simulink library "apm"  (R2021b)
settings: Solver=VariableStepAuto  StartTime=0.0  StopTime=10.0  RelTol=1e-3
settings Model: Creator=FVT22115  LastModifiedBy=FVT23010

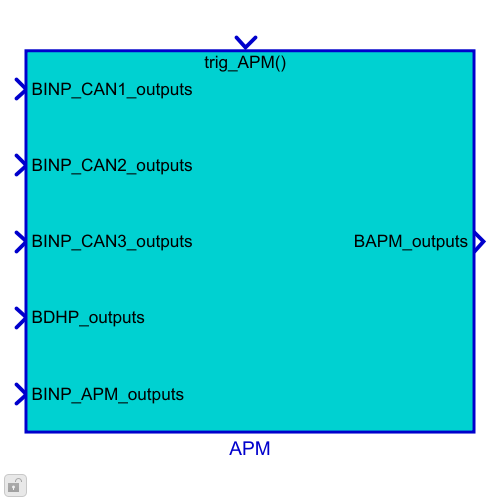
[thumbnail: Simulink's stored preview of the top-level diagram]
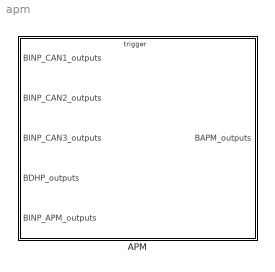
== system apm ==
  APM : Subsystem
      settings: RTWSystemCode=Nonreusable function  RTWFcnNameOpts=Use subsystem name  RTWFileNameOpts=Use subsystem name

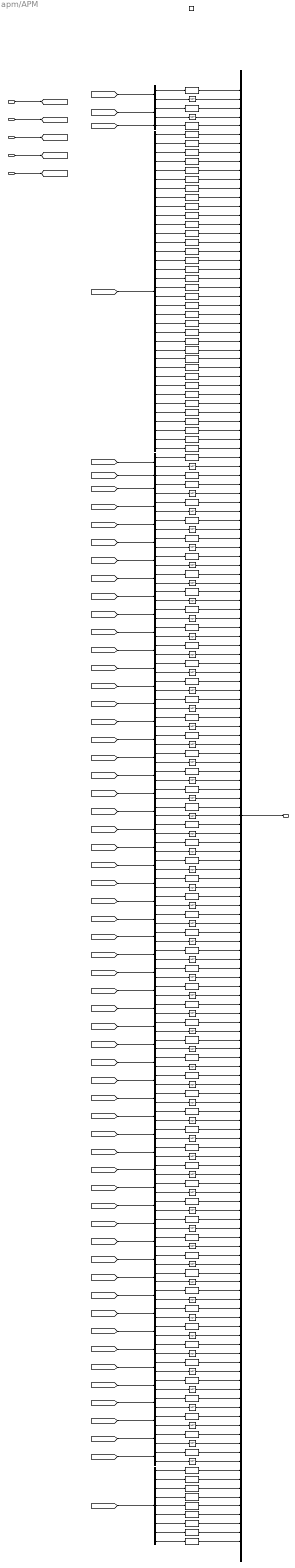
== system apm/APM ==
  BINP_CAN1_outputs : Inport  OutDataTypeStr=Bus: BINP_CAN1_outputs
  BINP_CAN2_outputs : Inport  Port=2  OutDataTypeStr=Bus: BINP_CAN2_outputs
  BINP_CAN3_outputs : Inport  Port=3  OutDataTypeStr=Bus: BINP_CAN3_outputs
  BDHP_outputs : Inport  Port=4  OutDataTypeStr=Bus: BDHP_outputs
  BINP_APM_outputs : Inport  Port=5  OutDataTypeStr=Bus: BINP_APM_outputs
  trig_APM : TriggerPort  TriggerType=function-call  VariantControl=(inherit)
  Bus Creator1 : BusCreator  Inputs=163  OutDataTypeStr=Bus: BAPM_outputs  NonVirtualBus=on
  Bus Selector : BusSelector  OutputSignals=VINP_FSOffSw_enum,VINP_CANMsgValidIVI2_flg
  Bus Selector1 : BusSelector  OutputSignals=VINP_PASDRMR_cm,VINP_PASDRML_cm,VINP_PASDRCR_cm,VINP_PASDRCL_cm,VINP_PASDFMR_cm,VINP_PASDFML_cm,VINP_PASDFCR_cm,VINP_PASDFCL_cm,VINP_APSDRLR_cm,VINP_APSDRLL_cm,VINP_APSDFLR_cm,VINP_APSDFLL_cm,VINP_PASAFCL_enum,VINP_PASARMR_enum,VINP_PASARML_enum,VINP_PASARCR_enum,VINP_PASARCL_enum,VINP_PASAFMR_enum,VINP_PASAFML_enum,VINP_PASAFCR_enum,VINP_USSStaRMR_flg,VINP_USSStaRML_flg,VINP_USSStaRLR_flg,VINP_USSStaRLL_flg,VINP_USSStaRCR_flg,VINP_USSStaRCL_flg,VINP_USSStaFMR_flg,VINP_USSStaFML_flg,VINP_USSStaFLR_flg,VINP_USSStaFLL_flg,VINP_USSStaFCR_flg,VINP_USSStaFCL_flg,VINP_Chime_enum,VINP_SNSRLayout_enum,VINP_StaFSya_flg,VINP_ModOperation_enum
  Bus Selector10 : BusSelector  OutputSignals=VINP_LFRawWhlSpeedV_flg,VINP_CANMsgValidESC1_flg
  Bus Selector11 : BusSelector  OutputSignals=VINP_RFRawWhlSpeedV_flg,VINP_CANMsgValidESC1_flg
  Bus Selector12 : BusSelector  OutputSignals=VINP_LRRawWhlSpeedV_flg,VINP_CANMsgValidESC1_flg
  Bus Selector13 : BusSelector  OutputSignals=VINP_RRRawWhlSpeedV_flg,VINP_CANMsgValidESC1_flg
  Bus Selector14 : BusSelector  OutputSignals=VINP_LFWhlRotDir_enum,VINP_CANMsgValidESC1_flg
  Bus Selector15 : BusSelector  OutputSignals=VINP_RFWhlRotDir_enum,VINP_CANMsgValidESC1_flg
  Bus Selector16 : BusSelector  OutputSignals=VINP_LRWhlRotDir_enum,VINP_CANMsgValidESC1_flg
  Bus Selector17 : BusSelector  OutputSignals=VINP_RRWhlRotDir_enum,VINP_CANMsgValidESC1_flg
  Bus Selector18 : BusSelector  OutputSignals=VINP_LFPulseCountV_flg,VINP_CANMsgValidESC1_flg
  Bus Selector19 : BusSelector  OutputSignals=VINP_RFPulseCountV_flg,VINP_CANMsgValidESC1_flg
  Bus Selector2 : BusSelector  OutputSignals=VINP_VehSpeed_kph,VINP_CANMsgValidESC1_flg
  Bus Selector20 : BusSelector  OutputSignals=VINP_LRPulseCountV_flg,VINP_CANMsgValidESC1_flg
  Bus Selector21 : BusSelector  OutputSignals=VINP_RRPulseCountV_flg,VINP_CANMsgValidESC1_flg
  Bus Selector22 : BusSelector  OutputSignals=VINP_LFPulseCount_enum,VINP_CANMsgValidESC1_flg
  Bus Selector23 : BusSelector  OutputSignals=VINP_RFPulseCount_enum,VINP_CANMsgValidESC1_flg
  Bus Selector24 : BusSelector  OutputSignals=VINP_LRPulseCount_enum,VINP_CANMsgValidESC1_flg
  Bus Selector25 : BusSelector  OutputSignals=VINP_RRPulseCount_enum,VINP_CANMsgValidESC1_flg
  Bus Selector26 : BusSelector  OutputSignals=VINP_ShifterHandleCmd_enum,VINP_CANMsgValidShifter1_flg
  Bus Selector27 : BusSelector  OutputSignals=VINP_DriIntend_enum,VINP_CANMsgValidEPS1_flg
  Bus Selector28 : BusSelector  OutputSignals=VINP_EPSAOIControl_enum,VINP_CANMsgValidEPS1_flg
  Bus Selector29 : BusSelector  OutputSignals=VINP_SASAngle_Deg,VINP_CANMsgValidEPS1_flg
  Bus Selector3 : BusSelector  OutputSignals=VINP_ChrgPlugSta_enum
  Bus Selector30 : BusSelector  OutputSignals=VINP_SASSpeed_degps,VINP_CANMsgValidEPS1_flg
  Bus Selector31 : BusSelector  OutputSignals=VINP_SASSpeedValid_flg,VINP_CANMsgValidEPS1_flg
  Bus Selector32 : BusSelector  OutputSignals=VINP_SASCAL_flg,VINP_CANMsgValidEPS1_flg
  Bus Selector33 : BusSelector  OutputSignals=VINP_SASV_flg,VINP_CANMsgValidEPS1_flg
  Bus Selector34 : BusSelector  OutputSignals=VINP_GRADE_Deg,VINP_CANMsgValidESC1_flg
  Bus Selector35 : BusSelector  OutputSignals=VINP_YawRate_degps,VINP_CANMsgValidESC5_flg
  Bus Selector36 : BusSelector  OutputSignals=VINP_LatAccel_Gps,VINP_CANMsgValidESC5_flg
  Bus Selector37 : BusSelector  OutputSignals=VINP_MCPressure_bar,VINP_CANMsgValidESC5_flg
  Bus Selector38 : BusSelector  OutputSignals=VINP_LongAccel_Gps,VINP_CANMsgValidESC5_flg
  Bus Selector39 : BusSelector  OutputSignals=VINP_YawRateV_flg,VINP_CANMsgValidESC5_flg
  Bus Selector4 : BusSelector  OutputSignals=VINP_BrkPedalPos_pct,VINP_CANMsgValidESC5_flg
  Bus Selector40 : BusSelector  OutputSignals=VINP_LatAccelV_flg,VINP_CANMsgValidESC5_flg
  Bus Selector41 : BusSelector  OutputSignals=VINP_LongAccelV_flg,VINP_CANMsgValidESC5_flg
  Bus Selector42 : BusSelector  OutputSignals=VINP_BrkSwSta_flg,VINP_CANMsgValidESC5_flg
  Bus Selector43 : BusSelector  OutputSignals=VINP_BrkSwV_flg,VINP_CANMsgValidESC5_flg
  Bus Selector44 : BusSelector  OutputSignals=VINP_ESCStandstill_flg,VINP_CANMsgValidESC5_flg
  Bus Selector45 : BusSelector  OutputSignals=VINP_ESCAPSSta_enum,VINP_CANMsgValidESC5_flg
  Bus Selector46 : BusSelector  OutputSignals=VINP_EPBExtReleaseAvail_flg,VINP_CANMsgValidEPB1_flg
  Bus Selector47 : BusSelector  OutputSignals=VINP_EPBExtApplyAvail_flg,VINP_CANMsgValidEPB1_flg
  Bus Selector48 : BusSelector  OutputSignals=VINP_EPBErrSta_enum,VINP_CANMsgValidEPB1_flg
  Bus Selector49 : BusSelector  OutputSignals=VINP_AVMparkingcancel_enum,VINP_CANMsgValidIVI2_flg
  Bus Selector5 : BusSelector  OutputSignals=VDHP_ActAPSPosn_pct
  Bus Selector50 : BusSelector  OutputSignals=VINP_AVMparkingexcute_enum,VINP_CANMsgValidIVI2_flg
  Bus Selector51 : BusSelector  OutputSignals=VINP_AVMParkingmode_enum,VINP_CANMsgValidIVI2_flg
  Bus Selector52 : BusSelector  OutputSignals=VINP_EPBSta_enum,VINP_CANMsgValidEPB1_flg
  Bus Selector53 : BusSelector  OutputSignals=VINP_AVMErrSTA_flg,VINP_CANMsgValidIVI2_flg
  Bus Selector54 : BusSelector  OutputSignals=VINP_IVIStatus_flg,VINP_CANMsgValidIVI2_flg
  Bus Selector55 : BusSelector  OutputSignals=VINP_CAASSw_enum,VINP_CANMsgValidIVI2_flg
  Bus Selector56 : BusSelector  OutputSignals=VINP_IVIScreen_enum,VINP_CANMsgValidIVI2_flg
  Bus Selector57 : BusSelector  OutputSignals=VINP_APSProgressPCT_pct,VINP_APSRQDisplay_enum,VINP_APSSWVer_enum,VINP_APSHWVer_enum,VINP_APSExitCondition_enum,VINP_APSAngleTarget_Deg,VINP_APSVRqEPASCtrl_flg,VINP_APSRqEPASCtrl_flg,VINP_CAASSta_enum
  Bus Selector58 : BusSelector  OutputSignals=VINP_MCPressureV_flg,VINP_CANMsgValidESC5_flg
  Bus Selector59 : BusSelector  OutputSignals=VINP_ABSActive_flg,VINP_CANMsgValidESC1_flg
  Bus Selector6 : BusSelector  OutputSignals=VINP_LFRawWhlSpeed_kph,VINP_CANMsgValidESC1_flg
  Bus Selector61 : BusSelector  OutputSignals=VINP_TCSActive_flg,VINP_CANMsgValidESC1_flg
  Bus Selector62 : BusSelector  OutputSignals=VINP_DriverSeatBeltCmd_flg,VINP_CANMsgValidABM1_flg
  Bus Selector7 : BusSelector  OutputSignals=VINP_RFRawWhlSpeed_kph,VINP_CANMsgValidESC1_flg
  Bus Selector8 : BusSelector  OutputSignals=VINP_LRRawWhlSpeed_kph,VINP_CANMsgValidESC1_flg
  Bus Selector9 : BusSelector  OutputSignals=VINP_RRRawWhlSpeed_kph,VINP_CANMsgValidESC1_flg
  Data Type Conversion{1..104,106} (105 alike) : DataTypeConversion
  Logical Operator{,1..57} (58 alike) : Logic  Operator=NOT  AllPortsSameDT=off  OutDataTypeStr=boolean
  BAPM_outputs : Outport  OutDataTypeStr=Bus: BAPM_outputs
  wires:
  [BINP_CAN2_outputs] -> Bus Selector/1
  [BINP_CAN1_outputs] -> Bus Selector2/1
  Bus Creator1/1 -> BAPM_outputs/1  "BAPM_outputs"
  Bus Selector2/2 -> Logical Operator/1  "<VINP_CANMsgValidESC1_flg>"
  Bus Selector/1 -> Data Type Conversion3/1  "<VINP_FSOffSw_enum>"
  Bus Selector/2 -> Logical Operator1/1  "<VINP_CANMsgValidIVI2_flg>"
  Bus Selector2/1 -> Data Type Conversion1/1  "<VINP_VehSpeed_kph>"
  Bus Selector1/1 -> Data Type Conversion5/1  "<VINP_PASDRMR_cm>"
  Bus Selector1/2 -> Data Type Conversion4/1  "<VINP_PASDRML_cm>"
  Bus Selector1/3 -> Data Type Conversion7/1  "<VINP_PASDRCR_cm>"
  Bus Selector1/4 -> Data Type Conversion6/1  "<VINP_PASDRCL_cm>"
  Bus Selector1/5 -> Data Type Conversion9/1  "<VINP_PASDFMR_cm>"
  Bus Selector1/6 -> Data Type Conversion8/1  "<VINP_PASDFML_cm>"
  Bus Selector1/7 -> Data Type Conversion11/1  "<VINP_PASDFCR_cm>"
  Bus Selector1/8 -> Data Type Conversion10/1  "<VINP_PASDFCL_cm>"
  Bus Selector1/9 -> Data Type Conversion13/1  "<VINP_APSDRLR_cm>"
  Bus Selector1/10 -> Data Type Conversion12/1  "<VINP_APSDRLL_cm>"
  Bus Selector1/11 -> Data Type Conversion15/1  "<VINP_APSDFLR_cm>"
  Bus Selector1/12 -> Data Type Conversion14/1  "<VINP_APSDFLL_cm>"
  Bus Selector1/13 -> Data Type Conversion17/1  "<VINP_PASAFCL_enum>"
  Bus Selector1/14 -> Data Type Conversion16/1  "<VINP_PASARMR_enum>"
  Bus Selector1/15 -> Data Type Conversion25/1  "<VINP_PASARML_enum>"
  Bus Selector1/16 -> Data Type Conversion24/1  "<VINP_PASARCR_enum>"
  Bus Selector1/17 -> Data Type Conversion27/1  "<VINP_PASARCL_enum>"
  Bus Selector1/18 -> Data Type Conversion26/1  "<VINP_PASAFMR_enum>"
  Bus Selector1/19 -> Data Type Conversion29/1  "<VINP_PASAFML_enum>"
  Bus Selector1/20 -> Data Type Conversion28/1  "<VINP_PASAFCR_enum>"
  Bus Selector1/21 -> Data Type Conversion31/1  "<VINP_USSStaRMR_flg>"
  Bus Selector1/22 -> Data Type Conversion30/1  "<VINP_USSStaRML_flg>"
  Bus Selector1/23 -> Data Type Conversion19/1  "<VINP_USSStaRLR_flg>"
  Bus Selector1/24 -> Data Type Conversion18/1  "<VINP_USSStaRLL_flg>"
  Bus Selector1/25 -> Data Type Conversion21/1  "<VINP_USSStaRCR_flg>"
  Bus Selector1/26 -> Data Type Conversion20/1  "<VINP_USSStaRCL_flg>"
  Bus Selector1/27 -> Data Type Conversion23/1  "<VINP_USSStaFMR_flg>"
  Bus Selector1/28 -> Data Type Conversion22/1  "<VINP_USSStaFML_flg>"
  Bus Selector1/29 -> Data Type Conversion39/1  "<VINP_USSStaFLR_flg>"
  Bus Selector1/30 -> Data Type Conversion38/1  "<VINP_USSStaFLL_flg>"
  Bus Selector1/31 -> Data Type Conversion33/1  "<VINP_USSStaFCR_flg>"
  Bus Selector1/32 -> Data Type Conversion32/1  "<VINP_USSStaFCL_flg>"
  Bus Selector1/33 -> Data Type Conversion35/1  "<VINP_Chime_enum>"
  Bus Selector1/34 -> Data Type Conversion34/1  "<VINP_SNSRLayout_enum>"
  Bus Selector1/35 -> Data Type Conversion37/1  "<VINP_StaFSya_flg>"
  Bus Selector1/36 -> Data Type Conversion36/1  "<VINP_ModOperation_enum>"
  Data Type Conversion1/1 -> Bus Creator1/1  "VAPM_VehSpeed_kph"
  Logical Operator/1 -> Bus Creator1/2  "VAPM_VehSpeedTimeOut_flg"
  Data Type Conversion3/1 -> Bus Creator1/3  "VAPM_FSOffSw_enum"
  Logical Operator1/1 -> Bus Creator1/4  "VAPM_FSOffSwTimeOut_flg"
  Bus Selector3/1 -> Data Type Conversion2/1  "<VINP_ChrgPlugSta_enum>"
  Data Type Conversion2/1 -> Bus Creator1/5  "VAPM_ChrgPlugSta_enum"
  BINP_CAN1_outputs/1 -> [BINP_CAN1_outputs]  "BINP_CAN1_outputs"
  BINP_CAN2_outputs/1 -> [BINP_CAN2_outputs]  "BINP_CAN2_outputs"
  BINP_CAN3_outputs/1 -> [BINP_CAN3_outputs]  "BINP_CAN3_outputs"
  [BINP_CAN1_outputs] -> Bus Selector4/1
  Bus Selector4/1 -> Data Type Conversion40/1  "<VINP_BrkPedalPos_pct>"
  Bus Selector4/2 -> Logical Operator2/1  "<VINP_CANMsgValidESC5_flg>"
  [BDHP_outputs] -> Bus Selector5/1
  BDHP_outputs/1 -> [BDHP_outputs]  "BDHP_outputs"
  Bus Selector6/1 -> Data Type Conversion42/1  "<VINP_LFRawWhlSpeed_kph>"
  [BINP_CAN1_outputs] -> Bus Selector6/1
  Bus Selector6/2 -> Logical Operator3/1  "<VINP_CANMsgValidESC1_flg>"
  Bus Selector7/2 -> Logical Operator4/1  "<VINP_CANMsgValidESC1_flg>"
  [BINP_CAN1_outputs] -> Bus Selector7/1
  Bus Selector7/1 -> Data Type Conversion43/1  "<VINP_RFRawWhlSpeed_kph>"
  Bus Selector8/1 -> Data Type Conversion44/1  "<VINP_LRRawWhlSpeed_kph>"
  [BINP_CAN1_outputs] -> Bus Selector8/1
  Bus Selector8/2 -> Logical Operator5/1  "<VINP_CANMsgValidESC1_flg>"
  Bus Selector9/2 -> Logical Operator6/1  "<VINP_CANMsgValidESC1_flg>"
  [BINP_CAN1_outputs] -> Bus Selector9/1
  Bus Selector9/1 -> Data Type Conversion45/1  "<VINP_RRRawWhlSpeed_kph>"
  [BINP_CAN1_outputs] -> Bus Selector13/1
  [BINP_CAN1_outputs] -> Bus Selector12/1
  [BINP_CAN1_outputs] -> Bus Selector11/1
  [BINP_CAN1_outputs] -> Bus Selector10/1
  Bus Selector14/1 -> Data Type Conversion50/1  "<VINP_LFWhlRotDir_enum>"
  [BINP_CAN1_outputs] -> Bus Selector14/1
  Bus Selector14/2 -> Logical Operator12/1  "<VINP_CANMsgValidESC1_flg>"
  Bus Selector15/2 -> Logical Operator13/1  "<VINP_CANMsgValidESC1_flg>"
  [BINP_CAN1_outputs] -> Bus Selector15/1
  Bus Selector15/1 -> Data Type Conversion51/1  "<VINP_RFWhlRotDir_enum>"
  Bus Selector16/1 -> Data Type Conversion52/1  "<VINP_LRWhlRotDir_enum>"
  [BINP_CAN1_outputs] -> Bus Selector16/1
  Bus Selector16/2 -> Logical Operator14/1  "<VINP_CANMsgValidESC1_flg>"
  Bus Selector17/2 -> Logical Operator11/1  "<VINP_CANMsgValidESC1_flg>"
  [BINP_CAN1_outputs] -> Bus Selector17/1
  Bus Selector17/1 -> Data Type Conversion53/1  "<VINP_RRWhlRotDir_enum>"
  Bus Selector21/1 -> Data Type Conversion57/1  "<VINP_RRPulseCountV_flg>"
  [BINP_CAN1_outputs] -> Bus Selector21/1
  Bus Selector21/2 -> Logical Operator15/1  "<VINP_CANMsgValidESC1_flg>"
  Bus Selector20/2 -> Logical Operator18/1  "<VINP_CANMsgValidESC1_flg>"
  [BINP_CAN1_outputs] -> Bus Selector20/1
  Bus Selector20/1 -> Data Type Conversion56/1  "<VINP_LRPulseCountV_flg>"
  Bus Selector19/1 -> Data Type Conversion55/1  "<VINP_RFPulseCountV_flg>"
  [BINP_CAN1_outputs] -> Bus Selector19/1
  Bus Selector19/2 -> Logical Operator17/1  "<VINP_CANMsgValidESC1_flg>"
  Bus Selector18/2 -> Logical Operator16/1  "<VINP_CANMsgValidESC1_flg>"
  [BINP_CAN1_outputs] -> Bus Selector18/1
  Bus Selector18/1 -> Data Type Conversion54/1  "<VINP_LFPulseCountV_flg>"
  Bus Selector5/1 -> Data Type Conversion41/1  "<VDHP_ActAPSPosn_pct>"
  [BINP_CAN3_outputs] -> Bus Selector3/1
  Data Type Conversion5/1 -> Bus Creator1/6  "VAPM_PASDRMR_cm"
  Data Type Conversion4/1 -> Bus Creator1/7  "VAPM_PASDRML_cm"
  Data Type Conversion7/1 -> Bus Creator1/8  "VAPM_PASDRCR_cm"
  Data Type Conversion6/1 -> Bus Creator1/9  "VAPM_PASDRCL_cm"
  Data Type Conversion9/1 -> Bus Creator1/10  "VAPM_PASDFMR_cm"
  Data Type Conversion8/1 -> Bus Creator1/11  "VAPM_PASDFML_cm"
  Data Type Conversion11/1 -> Bus Creator1/12  "VAPM_PASDFCR_cm"
  Data Type Conversion10/1 -> Bus Creator1/13  "VAPM_PASDFCL_cm"
  Data Type Conversion13/1 -> Bus Creator1/14  "VAPM_APSDRLR_cm"
  Data Type Conversion12/1 -> Bus Creator1/15  "VAPM_APSDRLL_cm"
  Data Type Conversion15/1 -> Bus Creator1/16  "VAPM_APSDFLR_cm"
  Data Type Conversion14/1 -> Bus Creator1/17  "VAPM_APSDFLL_cm"
  Data Type Conversion17/1 -> Bus Creator1/18  "VAPM_PASAFCL_enum"
  Data Type Conversion16/1 -> Bus Creator1/19  "VAPM_PASARMR_enum"
  Data Type Conversion25/1 -> Bus Creator1/20  "VAPM_PASARML_enum"
  Data Type Conversion24/1 -> Bus Creator1/21  "VAPM_PASARCR_enum"
  Data Type Conversion27/1 -> Bus Creator1/22  "VAPM_PASARCL_enum"
  Data Type Conversion26/1 -> Bus Creator1/23  "VAPM_PASAFMR_enum"
  Data Type Conversion29/1 -> Bus Creator1/24  "VAPM_PASAFML_enum"
  Data Type Conversion28/1 -> Bus Creator1/25  "VAPM_PASAFCR_enum"
  Data Type Conversion31/1 -> Bus Creator1/26  "VAPM_USSStaRMR_flg"
  Data Type Conversion30/1 -> Bus Creator1/27  "VAPM_USSStaRML_flg"
  Data Type Conversion19/1 -> Bus Creator1/28  "VAPM_USSStaRLR_flg"
  Data Type Conversion18/1 -> Bus Creator1/29  "VAPM_USSStaRLL_flg"
  Data Type Conversion21/1 -> Bus Creator1/30  "VAPM_USSStaRCR_flg"
  Data Type Conversion20/1 -> Bus Creator1/31  "VAPM_USSStaRCL_flg"
  Data Type Conversion23/1 -> Bus Creator1/32  "VAPM_USSStaFMR_flg"
  Data Type Conversion22/1 -> Bus Creator1/33  "VAPM_USSStaFML_flg"
  Data Type Conversion39/1 -> Bus Creator1/34  "VAPM_USSStaFLR_flg"
  Data Type Conversion38/1 -> Bus Creator1/35  "VAPM_USSStaFLL_flg"
  Data Type Conversion33/1 -> Bus Creator1/36  "VAPM_USSStaFCR_flg"
  Data Type Conversion32/1 -> Bus Creator1/37  "VAPM_USSStaFCL_flg"
  Data Type Conversion35/1 -> Bus Creator1/38  "VAPM_Chime_enum"
  Data Type Conversion34/1 -> Bus Creator1/39  "VAPM_SNSRLayout_enum"
  Data Type Conversion37/1 -> Bus Creator1/40  "VAPM_StaFSya_flg"
  Data Type Conversion36/1 -> Bus Creator1/41  "VAPM_ModOperation_enum"
  Data Type Conversion40/1 -> Bus Creator1/42  "VAPM_BrkPedalPos_pct"
  Data Type Conversion41/1 -> Bus Creator1/44  "VAPM_ActAPSPosn_pct"
  Data Type Conversion42/1 -> Bus Creator1/45  "VAPM_LFRawWhlSpeed_kph"
  Data Type Conversion43/1 -> Bus Creator1/47  "VAPM_RFRawWhlSpeed_kph"
  Data Type Conversion44/1 -> Bus Creator1/49  "VAPM_LRRawWhlSpeed_kph"
  Data Type Conversion45/1 -> Bus Creator1/51  "VAPM_RRRawWhlSpeed_kph"
  Data Type Conversion46/1 -> Bus Creator1/53  "VAPM_LFRawWhlSpeedV_flg"
  Data Type Conversion47/1 -> Bus Creator1/55  "VAPM_RFRawWhlSpeedV_flg"
  Data Type Conversion48/1 -> Bus Creator1/57  "VAPM_LRRawWhlSpeedV_flg"
  Data Type Conversion49/1 -> Bus Creator1/59  "VAPM_RRRawWhlSpeedV_flg"
  Data Type Conversion50/1 -> Bus Creator1/61  "VAPM_LFWhlRotDir_enum"
  Data Type Conversion51/1 -> Bus Creator1/63  "VAPM_RFWhlRotDir_enum"
  Data Type Conversion52/1 -> Bus Creator1/65  "VAPM_LRWhlRotDir_enum"
  Data Type Conversion53/1 -> Bus Creator1/67  "VAPM_RRWhlRotDir_enum"
  Data Type Conversion54/1 -> Bus Creator1/69  "VAPM_LFPulseCountV_flg"
  Data Type Conversion55/1 -> Bus Creator1/71  "VAPM_RFPulseCountV_flg"
  Data Type Conversion56/1 -> Bus Creator1/73  "VAPM_LRPulseCountV_flg"
  Data Type Conversion57/1 -> Bus Creator1/75  "VAPM_RRPulseCountV_flg"
  Logical Operator2/1 -> Bus Creator1/43  "VAPM_BrkPedalPosTimeOut_flg"
  Logical Operator3/1 -> Bus Creator1/46  "VAPM_LFRawWhlSpeedTimeOut_flg"
  Logical Operator4/1 -> Bus Creator1/48  "VAPM_RFRawWhlSpeedTimeOut_flg"
  Logical Operator5/1 -> Bus Creator1/50  "VAPM_LRRawWhlSpeedTimeOut_flg"
  Logical Operator6/1 -> Bus Creator1/52  "VAPM_RRRawWhlSpeedTimeOut_flg"
  Logical Operator7/1 -> Bus Creator1/54  "VAPM_LFRawWhlSpeedVTimeOut_flg"
  Logical Operator8/1 -> Bus Creator1/56  "VAPM_RFRawWhlSpeedVTimeOut_flg"
  Logical Operator9/1 -> Bus Creator1/58  "VAPM_LRRawWhlSpeedVTimeOut_flg"
  Logical Operator10/1 -> Bus Creator1/60  "VAPM_RRRawWhlSpeedVTimeOut_flg"
  Logical Operator12/1 -> Bus Creator1/62  "VAPM_LFWhlRotDirTimeOut_flg"
  Logical Operator13/1 -> Bus Creator1/64  "VAPM_RFWhlRotDirTimeOut_flg"
  Logical Operator14/1 -> Bus Creator1/66  "VAPM_LRWhlRotDirTimeOut_flg"
  Logical Operator11/1 -> Bus Creator1/68  "VAPM_RRWhlRotDirTimeOut_flg"
  Logical Operator16/1 -> Bus Creator1/70  "VAPM_LFPulseCountVTimeOut_flg"
  Logical Operator17/1 -> Bus Creator1/72  "VAPM_RFPulseCountVTimeOut_flg"
  Logical Operator18/1 -> Bus Creator1/74  "VAPM_LRPulseCountVTimeOut_flg"
  Logical Operator15/1 -> Bus Creator1/76  "VAPM_RRPulseCountVTimeOut_flg"
  Logical Operator19/1 -> Bus Creator1/84  "VAPM_RRPulseCountTimeOut_flg"
  Logical Operator22/1 -> Bus Creator1/82  "VAPM_LRPulseCountTimeOut_flg"
  Logical Operator21/1 -> Bus Creator1/80  "VAPM_RFPulseCountTimeOut_flg"
  Logical Operator20/1 -> Bus Creator1/78  "VAPM_LFPulseCountTimeOut_flg"
  Data Type Conversion61/1 -> Bus Creator1/83  "VAPM_RRPulseCount_enum"
  Data Type Conversion60/1 -> Bus Creator1/81  "VAPM_LRPulseCount_enum"
  Data Type Conversion59/1 -> Bus Creator1/79  "VAPM_RFPulseCount_enum"
  Data Type Conversion58/1 -> Bus Creator1/77  "VAPM_LFPulseCount_enum"
  Bus Selector22/1 -> Data Type Conversion58/1  "<VINP_LFPulseCount_enum>"
  [BINP_CAN1_outputs] -> Bus Selector22/1
  Bus Selector22/2 -> Logical Operator20/1  "<VINP_CANMsgValidESC1_flg>"
  Bus Selector23/2 -> Logical Operator21/1  "<VINP_CANMsgValidESC1_flg>"
  [BINP_CAN1_outputs] -> Bus Selector23/1
  Bus Selector23/1 -> Data Type Conversion59/1  "<VINP_RFPulseCount_enum>"
  Bus Selector24/1 -> Data Type Conversion60/1  "<VINP_LRPulseCount_enum>"
  [BINP_CAN1_outputs] -> Bus Selector24/1
  Bus Selector24/2 -> Logical Operator22/1  "<VINP_CANMsgValidESC1_flg>"
  Bus Selector25/2 -> Logical Operator19/1  "<VINP_CANMsgValidESC1_flg>"
  [BINP_CAN1_outputs] -> Bus Selector25/1
  Bus Selector25/1 -> Data Type Conversion61/1  "<VINP_RRPulseCount_enum>"
  [BINP_CAN3_outputs] -> Bus Selector26/1
  Bus Selector26/1 -> Data Type Conversion62/1  "<VINP_ShifterHandleCmd_enum>"
  Bus Selector26/2 -> Logical Operator23/1  "<VINP_CANMsgValidShifter1_flg>"
  Data Type Conversion62/1 -> Bus Creator1/85  "VAPM_ShifterHandleCmd_enum"
  Logical Operator23/1 -> Bus Creator1/86  "VAPM_ShifterHandleCmdTimeOut_flg"
  [BINP_CAN1_outputs] -> Bus Selector27/1
  [BINP_CAN1_outputs] -> Bus Selector28/1
  [BINP_CAN1_outputs] -> Bus Selector29/1
  Bus Selector29/1 -> Data Type Conversion65/1  "<VINP_SASAngle_Deg>"
  Bus Selector29/2 -> Logical Operator26/1  "<VINP_CANMsgValidEPS1_flg>"
  Bus Selector30/2 -> Logical Operator27/1  "<VINP_CANMsgValidEPS1_flg>"
  [BINP_CAN1_outputs] -> Bus Selector30/1
  [BINP_CAN1_outputs] -> Bus Selector31/1
  Bus Selector31/2 -> Logical Operator28/1  "<VINP_CANMsgValidEPS1_flg>"
  Data Type Conversion65/1 -> Bus Creator1/91  "VAPM_SASAngle_Deg"
  Logical Operator26/1 -> Bus Creator1/92  "VAPM_SASAngleTimeOut_flg"
  Bus Selector32/2 -> Logical Operator29/1  "<VINP_CANMsgValidEPS1_flg>"
  [BINP_CAN1_outputs] -> Bus Selector32/1
  [BINP_CAN1_outputs] -> Bus Selector33/1
  Bus Selector33/2 -> Logical Operator30/1  "<VINP_CANMsgValidEPS1_flg>"
  Logical Operator31/1 -> Bus Creator1/102  "VAPM_GRADETimeOut_flg"
  Data Type Conversion70/1 -> Bus Creator1/101  "VAPM_GRADE_Deg"
  Bus Selector34/2 -> Logical Operator31/1  "<VINP_CANMsgValidESC1_flg>"
  Bus Selector34/1 -> Data Type Conversion70/1  "<VINP_GRADE_Deg>"
  [BINP_CAN1_outputs] -> Bus Selector34/1
  [BINP_CAN1_outputs] -> Bus Selector35/1
  Bus Selector35/1 -> Data Type Conversion71/1  "<VINP_YawRate_degps>"
  Bus Selector35/2 -> Logical Operator32/1  "<VINP_CANMsgValidESC5_flg>"
  Data Type Conversion71/1 -> Bus Creator1/103  "VAPM_YawRate_degps"
  Logical Operator32/1 -> Bus Creator1/104  "VAPM_YawRateTimeOut_flg"
  Logical Operator33/1 -> Bus Creator1/106  "VAPM_LatAccelTimeOut_flg"
  Data Type Conversion72/1 -> Bus Creator1/105  "VAPM_LatAccel_Gps"
  Bus Selector36/2 -> Logical Operator33/1  "<VINP_CANMsgValidESC5_flg>"
  Bus Selector36/1 -> Data Type Conversion72/1  "<VINP_LatAccel_Gps>"
  [BINP_CAN1_outputs] -> Bus Selector36/1
  [BINP_CAN1_outputs] -> Bus Selector37/1
  Bus Selector37/1 -> Data Type Conversion73/1  "<VINP_MCPressure_bar>"
  Bus Selector37/2 -> Logical Operator34/1  "<VINP_CANMsgValidESC5_flg>"
  Bus Selector38/2 -> Logical Operator35/1  "<VINP_CANMsgValidESC5_flg>"
  Bus Selector38/1 -> Data Type Conversion74/1  "<VINP_LongAccel_Gps>"
  [BINP_CAN1_outputs] -> Bus Selector38/1
  Data Type Conversion74/1 -> Bus Creator1/107  "VAPM_LongAccel_Gps"
  Logical Operator35/1 -> Bus Creator1/108  "VAPM_LongAccelTimeOut_flg"
  Data Type Conversion73/1 -> Bus Creator1/109  "VAPM_MCPressure_bar"
  Logical Operator34/1 -> Bus Creator1/110  "VAPM_MCPressureTimeOut_flg"
  [BINP_CAN1_outputs] -> Bus Selector41/1
  Bus Selector41/2 -> Logical Operator38/1  "<VINP_CANMsgValidESC5_flg>"
  [BINP_CAN1_outputs] -> Bus Selector40/1
  Bus Selector40/2 -> Logical Operator37/1  "<VINP_CANMsgValidESC5_flg>"
  Bus Selector39/2 -> Logical Operator36/1  "<VINP_CANMsgValidESC5_flg>"
  [BINP_CAN1_outputs] -> Bus Selector39/1
  Bus Selector42/2 -> Logical Operator39/1  "<VINP_CANMsgValidESC5_flg>"
  [BINP_CAN1_outputs] -> Bus Selector42/1
  Bus Selector42/1 -> Data Type Conversion78/1  "<VINP_BrkSwSta_flg>"
  Data Type Conversion78/1 -> Bus Creator1/119  "VAPM_BrkSwSta_flg"
  Logical Operator39/1 -> Bus Creator1/120  "VAPM_BrkSwStaTimeOut_flg"
  Logical Operator40/1 -> Bus Creator1/122  "VAPM_BrkSwVTimeOut_flg"
  Data Type Conversion79/1 -> Bus Creator1/121  "VAPM_BrkSwV_flg"
  Bus Selector43/1 -> Data Type Conversion79/1  "<VINP_BrkSwV_flg>"
  [BINP_CAN1_outputs] -> Bus Selector43/1
  Bus Selector43/2 -> Logical Operator40/1  "<VINP_CANMsgValidESC5_flg>"
  [BINP_CAN1_outputs] -> Bus Selector44/1
  Bus Selector44/2 -> Logical Operator41/1  "<VINP_CANMsgValidESC5_flg>"
  Bus Selector45/2 -> Logical Operator42/1  "<VINP_CANMsgValidESC5_flg>"
  [BINP_CAN1_outputs] -> Bus Selector45/1
  [BINP_CAN1_outputs] -> Bus Selector47/1
  Bus Selector47/2 -> Logical Operator44/1  "<VINP_CANMsgValidEPB1_flg>"
  Bus Selector46/2 -> Logical Operator43/1  "<VINP_CANMsgValidEPB1_flg>"
  [BINP_CAN1_outputs] -> Bus Selector46/1
  Bus Selector48/2 -> Logical Operator45/1  "<VINP_CANMsgValidEPB1_flg>"
  [BINP_CAN1_outputs] -> Bus Selector48/1
  Bus Selector48/1 -> Data Type Conversion84/1  "<VINP_EPBErrSta_enum>"
  Data Type Conversion84/1 -> Bus Creator1/131  "VAPM_EPBErrSta_enum"
  Logical Operator45/1 -> Bus Creator1/132  "VAPM_EPBErrStaTimeOut_flg"
  Bus Selector49/2 -> Logical Operator46/1  "<VINP_CANMsgValidIVI2_flg>"
  [BINP_CAN2_outputs] -> Bus Selector49/1
  [BINP_CAN2_outputs] -> Bus Selector50/1
  Bus Selector50/2 -> Logical Operator47/1  "<VINP_CANMsgValidIVI2_flg>"
  Bus Selector51/2 -> Logical Operator48/1  "<VINP_CANMsgValidIVI2_flg>"
  [BINP_CAN2_outputs] -> Bus Selector51/1
  Logical Operator49/1 -> Bus Creator1/134  "VAPM_EPBStaTimeOut_flg"
  Data Type Conversion88/1 -> Bus Creator1/133  "VAPM_EPBSta_enum"
  Bus Selector52/1 -> Data Type Conversion88/1  "<VINP_EPBSta_enum>"
  [BINP_CAN1_outputs] -> Bus Selector52/1
  Bus Selector52/2 -> Logical Operator49/1  "<VINP_CANMsgValidEPB1_flg>"
  [BINP_CAN2_outputs] -> Bus Selector53/1
  Bus Selector53/2 -> Logical Operator50/1  "<VINP_CANMsgValidIVI2_flg>"
  Bus Selector54/2 -> Logical Operator51/1  "<VINP_CANMsgValidIVI2_flg>"
  [BINP_CAN2_outputs] -> Bus Selector54/1
  Bus Selector54/1 -> Data Type Conversion90/1  "<VINP_IVIStatus_flg>"
  Data Type Conversion90/1 -> Bus Creator1/143  "VAPM_IVIStatus_flg"
  Logical Operator51/1 -> Bus Creator1/144  "VAPM_IVIStatusTimeOut_flg"
  [BINP_CAN2_outputs] -> Bus Selector55/1
  Bus Selector55/2 -> Logical Operator52/1  "<VINP_CANMsgValidIVI2_flg>"
  Bus Selector56/2 -> Logical Operator53/1  "<VINP_CANMsgValidIVI2_flg>"
  [BINP_CAN2_outputs] -> Bus Selector56/1
  Logical Operator27/1 -> Bus Creator1/94  "VAPM_SASSpeedTimeOut_flg"
  Logical Operator24/1 -> Bus Creator1/88  "VAPM_DriIntendTimeOut_flg"
  Logical Operator25/1 -> Bus Creator1/90  "VAPM_EPSAOIControlTimeOut_flg"
  Logical Operator28/1 -> Bus Creator1/96  "VAPM_SASSpeedValidTimeOut_flg"
  Logical Operator29/1 -> Bus Creator1/98  "VAPM_SASCALTimeOut_flg"
  Logical Operator30/1 -> Bus Creator1/100  "VAPM_SASVTimeOut_flg"
  Logical Operator36/1 -> Bus Creator1/112  "VAPM_YawRateVTimeOut_flg"
  Logical Operator37/1 -> Bus Creator1/114  "VAPM_LatAccelVTimeOut_flg"
  Logical Operator38/1 -> Bus Creator1/116  "VAPM_LongAccelVTimeOut_flg"
  Logical Operator41/1 -> Bus Creator1/124  "VAPM_ESCStandstillTimeOut_flg"
  Logical Operator42/1 -> Bus Creator1/126  "VAPM_ESCAPSStaTimeOut_flg"
  Logical Operator43/1 -> Bus Creator1/128  "VAPM_EPBExtReleaseAvailTimeOut_flg"
  Logical Operator44/1 -> Bus Creator1/130  "VAPM_EPBExtApplyAvailTimeOut_flg"
  Logical Operator46/1 -> Bus Creator1/136  "VAPM_AVMparkingcancelTimeOut_flg"
  Logical Operator47/1 -> Bus Creator1/138  "VAPM_AVMparkingexcuteTimeOut_flg"
  Logical Operator48/1 -> Bus Creator1/140  "VAPM_AVMParkingmodeTimeOut_flg"
  Logical Operator50/1 -> Bus Creator1/142  "VAPM_AVMErrSTATimeOut_flg"
  Logical Operator52/1 -> Bus Creator1/146  "VAPM_CAASSwTimeOut_flg"
  Logical Operator53/1 -> Bus Creator1/148  "VAPM_IVIScreenTimeOut_flg"
  BINP_APM_outputs/1 -> [BINP_APM_outputs]  "BINP_APM_outputs"
  [BINP_APM_outputs] -> Bus Selector1/1
  [BINP_APM_outputs] -> Bus Selector57/1
  Bus Selector57/9 -> Data Type Conversion101/1  "<VINP_CAASSta_enum>"
  Bus Selector57/8 -> Data Type Conversion102/1  "<VINP_APSRqEPASCtrl_flg>"
  Bus Selector57/7 -> Data Type Conversion100/1  "<VINP_APSVRqEPASCtrl_flg>"
  Bus Selector57/6 -> Data Type Conversion98/1  "<VINP_APSAngleTarget_Deg>"
  Bus Selector57/5 -> Data Type Conversion97/1  "<VINP_APSExitCondition_enum>"
  Bus Selector57/4 -> Data Type Conversion96/1  "<VINP_APSHWVer_enum>"
  Bus Selector57/3 -> Data Type Conversion95/1  "<VINP_APSSWVer_enum>"
  Bus Selector57/2 -> Data Type Conversion94/1  "<VINP_APSRQDisplay_enum>"
  Bus Selector57/1 -> Data Type Conversion93/1  "<VINP_APSProgressPCT_pct>"
  Bus Selector27/1 -> Data Type Conversion63/1  "<VINP_DriIntend_enum>"
  Data Type Conversion63/1 -> Bus Creator1/87  "VAPM_DriIntend_enum"
  Bus Selector27/2 -> Logical Operator24/1  "<VINP_CANMsgValidEPS1_flg>"
  Bus Selector28/1 -> Data Type Conversion64/1  "<VINP_EPSAOIControl_enum>"
  Data Type Conversion64/1 -> Bus Creator1/89  "VAPM_EPSAOIControl_enum"
  Bus Selector30/1 -> Data Type Conversion66/1  "<VINP_SASSpeed_degps>"
  Data Type Conversion66/1 -> Bus Creator1/93  "VAPM_SASSpeed_degps"
  Bus Selector31/1 -> Data Type Conversion67/1  "<VINP_SASSpeedValid_flg>"
  Data Type Conversion67/1 -> Bus Creator1/95  "VAPM_SASSpeedValid_flg"
  Bus Selector32/1 -> Data Type Conversion68/1  "<VINP_SASCAL_flg>"
  Data Type Conversion68/1 -> Bus Creator1/97  "VAPM_SASCAL_flg"
  Bus Selector33/1 -> Data Type Conversion69/1  "<VINP_SASV_flg>"
  Data Type Conversion69/1 -> Bus Creator1/99  "VAPM_SASV_flg"
  Bus Selector39/1 -> Data Type Conversion75/1  "<VINP_YawRateV_flg>"
  Data Type Conversion75/1 -> Bus Creator1/111  "VAPM_YawRateV_flg"
  Bus Selector40/1 -> Data Type Conversion76/1  "<VINP_LatAccelV_flg>"
  Data Type Conversion76/1 -> Bus Creator1/113  "VAPM_LatAccelV_flg"
  Bus Selector41/1 -> Data Type Conversion77/1  "<VINP_LongAccelV_flg>"
  Data Type Conversion77/1 -> Bus Creator1/115  "VAPM_LongAccelV_flg"
  Bus Selector44/1 -> Data Type Conversion80/1  "<VINP_ESCStandstill_flg>"
  Data Type Conversion80/1 -> Bus Creator1/123  "VAPM_ESCStandstill_flg"
  Bus Selector45/1 -> Data Type Conversion81/1  "<VINP_ESCAPSSta_enum>"
  Data Type Conversion81/1 -> Bus Creator1/125  "VAPM_ESCAPSSta_enum"
  Bus Selector46/1 -> Data Type Conversion82/1  "<VINP_EPBExtReleaseAvail_flg>"
  Data Type Conversion82/1 -> Bus Creator1/127  "VAPM_EPBExtReleaseAvail_flg"
  Bus Selector47/1 -> Data Type Conversion83/1  "<VINP_EPBExtApplyAvail_flg>"
  Data Type Conversion83/1 -> Bus Creator1/129  "VAPM_EPBExtApplyAvail_flg"
  Bus Selector49/1 -> Data Type Conversion85/1  "<VINP_AVMparkingcancel_enum>"
  Data Type Conversion85/1 -> Bus Creator1/135  "VAPM_AVMparkingcancel_enum"
  Bus Selector50/1 -> Data Type Conversion86/1  "<VINP_AVMparkingexcute_enum>"
  Data Type Conversion86/1 -> Bus Creator1/137  "VAPM_AVMparkingexcute_enum"
  Bus Selector51/1 -> Data Type Conversion87/1  "<VINP_AVMParkingmode_enum>"
  Data Type Conversion87/1 -> Bus Creator1/139  "VAPM_AVMParkingmode_enum"
  Bus Selector53/1 -> Data Type Conversion89/1  "<VINP_AVMErrSTA_flg>"
  Data Type Conversion89/1 -> Bus Creator1/141  "VAPM_AVMErrSTA_flg"
  Bus Selector55/1 -> Data Type Conversion91/1  "<VINP_CAASSw_enum>"
  Data Type Conversion91/1 -> Bus Creator1/145  "VAPM_CAASSw_enum"
  Bus Selector56/1 -> Data Type Conversion92/1  "<VINP_IVIScreen_enum>"
  Data Type Conversion92/1 -> Bus Creator1/147  "VAPM_IVIScreen_enum"
  Bus Selector10/1 -> Data Type Conversion46/1  "<VINP_LFRawWhlSpeedV_flg>"
  Bus Selector10/2 -> Logical Operator7/1  "<VINP_CANMsgValidESC1_flg>"
  Bus Selector11/1 -> Data Type Conversion47/1  "<VINP_RFRawWhlSpeedV_flg>"
  Bus Selector11/2 -> Logical Operator8/1  "<VINP_CANMsgValidESC1_flg>"
  Bus Selector12/1 -> Data Type Conversion48/1  "<VINP_LRRawWhlSpeedV_flg>"
  Bus Selector12/2 -> Logical Operator9/1  "<VINP_CANMsgValidESC1_flg>"
  Bus Selector13/1 -> Data Type Conversion49/1  "<VINP_RRRawWhlSpeedV_flg>"
  Bus Selector13/2 -> Logical Operator10/1  "<VINP_CANMsgValidESC1_flg>"
  Bus Selector58/1 -> Data Type Conversion106/1  "<VINP_MCPressureV_flg>"
  [BINP_CAN1_outputs] -> Bus Selector58/1
  Bus Selector58/2 -> Logical Operator54/1  "<VINP_CANMsgValidESC5_flg>"
  Logical Operator54/1 -> Bus Creator1/118  "VAPM_MCPressureVTimeOut_flg"
  Data Type Conversion106/1 -> Bus Creator1/117  "VAPM_MCPressureV_bar"
  [BINP_CAN1_outputs] -> Bus Selector59/1
  Bus Selector59/1 -> Data Type Conversion99/1  "<VINP_ABSActive_flg>"
  Bus Selector59/2 -> Logical Operator55/1  "<VINP_CANMsgValidESC1_flg>"
  Data Type Conversion99/1 -> Bus Creator1/149  "VAPM_ABSActive_flg"
  Logical Operator55/1 -> Bus Creator1/150  "VAPM_ABSActiveTimeOut_flg"
  Bus Selector61/1 -> Data Type Conversion103/1  "<VINP_TCSActive_flg>"
  Bus Selector61/2 -> Logical Operator56/1  "<VINP_CANMsgValidESC1_flg>"
  [BINP_CAN1_outputs] -> Bus Selector61/1
  [BINP_CAN1_outputs] -> Bus Selector62/1
  Bus Selector62/1 -> Data Type Conversion104/1  "<VINP_DriverSeatBeltCmd_flg>"
  Bus Selector62/2 -> Logical Operator57/1  "<VINP_CANMsgValidABM1_flg>"
  Logical Operator56/1 -> Bus Creator1/152  "VAPM_TCSActiveTimeOut_flg"
  Data Type Conversion103/1 -> Bus Creator1/151  "VAPM_TCSActive_flg"
  Data Type Conversion104/1 -> Bus Creator1/153  "VAPM_DriverSeatBeltCmd_flg"
  Logical Operator57/1 -> Bus Creator1/154  "VAPM_DriverSeatBeltCmdTimeOut_flg"
  Data Type Conversion93/1 -> Bus Creator1/155  "VAPM_APSProgressPCT_pct"
  Data Type Conversion94/1 -> Bus Creator1/156  "VAPM_APSRQDisplay_enum"
  Data Type Conversion95/1 -> Bus Creator1/157  "VAPM_APSSWVer_enum"
  Data Type Conversion96/1 -> Bus Creator1/158  "VAPM_APSHWVer_enum"
  Data Type Conversion97/1 -> Bus Creator1/159  "VAPM_APSExitCondition_enum"
  Data Type Conversion98/1 -> Bus Creator1/160  "VAPM_APSAngleTarget_Deg"
  Data Type Conversion100/1 -> Bus Creator1/161  "VAPM_APSVRqEPASCtrl_flg"
  Data Type Conversion102/1 -> Bus Creator1/162  "VAPM_APSRqEPASCtrl_flg"
  Data Type Conversion101/1 -> Bus Creator1/163  "VAPM_CAASSta_enum"
  Bus Selector28/2 -> Logical Operator25/1  "<VINP_CANMsgValidEPS1_flg>"
